simulink model "BaseEngineController_LS"  (Simulink 7.7)
settings: Solver=FixedStepDiscrete  StartTime=0.0  StopTime=10.0  RelTol=1e-3
PreLoadFcn:
  | try, eval([bdroot '_setup']); catch, eval('model_setup', ''); end
InitFcn:
  | try, eval([bdroot '_setup']); catch, eval('model_setup', ''); end
undefined symbols (not defined in the file): ECU555, High, motohawk_build_version, motohawk_trunc_name, motohawk_vardec_config_group, motohawk_vardec_path, True
libraries: MotoHawk_lib x1418, motohawk_control_primitives_lib x183, motohawk_engine_lib x32, simulink x21, motohawk_annotations_lib x9, AutoDoc_lib x8, simulink_extras x4, motohawk_ccp_examples_lib x1, motohawk_control_primitives_motoshare_lib x1
(part 18 of 27)

== system BaseEngineController_LS/Foreground/Inputs/PotentiometerSensors/APP2ForcedAdapt/Function-Call Subsystem ==
  function : TriggerPort  TriggerType=function-call
  First Time : motohawk_control_primitives_lib/First Time  SystemSampleTime=-1
  Logical Operator : Logic  Operator=OR  AllPortsSameDT=off  OutDataTypeStr=boolean
  motohawk_calibration : MotoHawk_lib/Calibration & Probing Blocks/motohawk_calibration  nam='APP2_AlwaysAdapt'  val=0  storage=Calibration  show_more=on  name_source=Use Parameter  data_type=boolean  read_level=1  write_level=1  ovr_cals=on  view_as=Enumeration  enum_struct={'Disabled', 'Enabled'}  vector_style=Wide Row  use_help_units=off  help=''  units=''  use_header_enum=off  row_header_enum={}  col_header_enum={}  use_min_max=off  min_val=-inf  max_val=inf  use_precision=off  precision=''  gain=1  offset=0  exp=1  use_mototune_group=off  mototune_group=motohawk_vardec_path(gcb)
  Out1 : Outport  InitialOutput=false
  wires:
  First Time/1 -> Logical Operator/1
  motohawk_calibration/1 -> Logical Operator/2
  Logical Operator/1 -> Out1/1

== system BaseEngineController_LS/Foreground/Outputs/AEM Infinity Dash/Dash Message 1/RPM_Filt ==
  Raw : Inport
  Constant : Constant
  First Order Low Pass (Tunable) : motohawk_control_primitives_lib/First Order Low Pass (Tunable)  SystemSampleTime=-1  nam='RPMFilt_LowPass'  samp_time=-1  group=motohawk_vardec_path(gcb)
  MinMax : MinMax  Function=max  Inputs=2
  Product : Product  Inputs=*/  RndMeth=Zero
  Product1 : Product  RndMeth=Zero
  Rounding Function : Rounding  Operator=round
  Switch : Switch  Threshold=1
  motohawk_calibration : MotoHawk_lib/Calibration & Probing Blocks/motohawk_calibration  nam='RPMFilt_Enable'  val=0  storage=Calibration  show_more=on  name_source=Use Parameter  data_type=uint8  read_level=1  write_level=1  ovr_cals=on  view_as=Enumeration  enum_struct={'Disabled', 'Enabled'}  vector_style=Wide Row  use_help_units=off  help=''  units=''  use_header_enum=off  row_header_enum={}  col_header_enum={}  use_min_max=off  min_val=-inf  max_val=inf  use_precision=off  precision=''  gain=1  offset=0  exp=1  use_mototune_group=off  mototune_group=motohawk_vardec_path(gcb)
  motohawk_calibration1 : MotoHawk_lib/Calibration & Probing Blocks/motohawk_calibration  nam='RPMFilt_RoundValue'  val=10  storage=Calibration  show_more=on  name_source=Use Parameter  data_type=uint16  read_level=1  write_level=1  ovr_cals=on  view_as=Number  enum_struct={'Disabled', 'Enabled'}  vector_style=Wide Row  use_help_units=on  help='RPM round value'  units='RPM'  use_header_enum=off  row_header_enum={}  col_header_enum={}  use_min_max=on  min_val=0  max_val=1000  use_precision=off  precision=''  gain=1  offset=0  exp=1  use_mototune_group=off  mototune_group=motohawk_vardec_path(gcb)
  motohawk_probe : MotoHawk_lib/Calibration & Probing Blocks/motohawk_probe  nam='RPMFilt_Final'  show_more=off  name_source=Use Parameter  read_level=1  view_as=Number  enum_struct={'Disabled', 'Enabled'}  vector_style=Wide Row  use_help_units=off  help=''  units=''  use_header_enum=off  row_header_enum={}  col_header_enum={}  use_precision=off  precision=''  gain=1  offset=0  exp=1  use_mototune_group=off  mototune_group=motohawk_vardec_path(gcb)
  motohawk_probe1 : MotoHawk_lib/Calibration & Probing Blocks/motohawk_probe  nam='RPMFilt_PostLowPass'  show_more=off  name_source=Use Parameter  read_level=1  view_as=Number  enum_struct={'Disabled', 'Enabled'}  vector_style=Wide Row  use_help_units=off  help=''  units=''  use_header_enum=off  row_header_enum={}  col_header_enum={}  use_precision=off  precision=''  gain=1  offset=0  exp=1  use_mototune_group=off  mototune_group=motohawk_vardec_path(gcb)
  Filt : Outport
  wires:
  Switch/1 -> Filt/1, motohawk_probe/1
  Raw/1 -> Switch/3, [RPM]
  motohawk_calibration/1 -> Switch/2
  Constant/1 -> MinMax/2
  motohawk_calibration1/1 -> MinMax/1
  MinMax/1 -> Product/2, Product1/2
  Product/1 -> Rounding Function/1
  Rounding Function/1 -> Product1/1
  Product1/1 -> Switch/1
  [RPM] -> First Order Low Pass (Tunable)/1
  First Order Low Pass (Tunable)/1 -> Product/1, motohawk_probe1/1

== system BaseEngineController_LS/Foreground/Outputs/AEM Infinity Dash/Dash Message 2/PHI_Filt ==
  PHI RAW : Inport
  PHI DR : Inport  Port=2
  Constant : Constant
  DecreasingFilter : Subsystem  TreatAsAtomicUnit=on
  First Order Low Pass : motohawk_control_primitives_lib/First Order Low Pass  SystemSampleTime=-1
  IncreasingFilter : Subsystem  TreatAsAtomicUnit=on
  Merge : Merge
  MinMax : MinMax  Function=max  Inputs=2  SaturateOnIntegerOverflow=on  InputSameDT=on
  Product : Product  Inputs=*/  SaturateOnIntegerOverflow=on  InputSameDT=on  OutDataTypeStr=Inherit: Same as first input
  Relational Operator3 : RelationalOperator  Operator=>  OutDataTypeStr=boolean
  Relational Operator4 : RelationalOperator  Operator=<  OutDataTypeStr=boolean
  Switch : Switch  Threshold=1
  Switch1 : Switch  Threshold=1
  Unit Delay{1..5} (5 alike) : UnitDelay  SampleTime=-1
  motohawk_calibration : MotoHawk_lib/Calibration & Probing Blocks/motohawk_calibration  nam='PHI1_DefaultVal'  val=0.5  storage=Calibration  show_more=off  name_source=Use Parameter  data_type=Inherit from 'Default Value'  read_level=1  write_level=1  ovr_cals=on  view_as=Number  enum_struct={'Disabled', 'Enabled'}  vector_style=Wide Row  use_help_units=off  help=''  units=''  use_header_enum=off  row_header_enum={}  col_header_enum={}  use_min_max=off  min_val=-inf  max_val=inf  use_precision=off  precision=''  gain=1  offset=0  exp=1  use_mototune_group=off  mototune_group=motohawk_vardec_path(gcb)
  motohawk_delta_time : MotoHawk_lib/Extra Development Blocks/motohawk_delta_time  samp_time=.005  init_val=.005  mode=Seconds (double)
  motohawk_probe : MotoHawk_lib/Calibration & Probing Blocks/motohawk_probe  nam='PHI1_FiltFin'  show_more=off  name_source=Use Parameter  read_level=1  view_as=Number  enum_struct={'Disabled', 'Enabled'}  vector_style=Wide Row  use_help_units=off  help=''  units=''  use_header_enum=off  row_header_enum={}  col_header_enum={}  use_precision=off  precision=''  gain=1  offset=0  exp=1  use_mototune_group=off  mototune_group=motohawk_vardec_path(gcb)
  Filt Out : Outport
  wires:
  PHI DR/1 -> Unit Delay5/1
  motohawk_calibration/1 -> Switch/3
  Unit Delay4/1 -> Unit Delay3/1
  Unit Delay3/1 -> Unit Delay1/1
  Unit Delay1/1 -> Unit Delay2/1
  Unit Delay2/1 -> Relational Operator4/1, Relational Operator3/1
  motohawk_delta_time/1 -> MinMax/1, Product/1
  MinMax/1 -> Product/2
  Merge/1 -> MinMax/2
  Relational Operator4/1 -> IncreasingFilter/Enable
  Relational Operator3/1 -> DecreasingFilter/Enable
  DecreasingFilter/1(Out1) -> Merge/2
  IncreasingFilter/1(Out1) -> Merge/1
  PHI RAW/1 -> First Order Low Pass/1, Unit Delay4/1, Relational Operator3/2, Relational Operator4/2
  [PHI_DR] -> Switch1/2
  Product/1 -> Switch1/1
  Constant/1 -> Switch1/3
  Switch1/1 -> First Order Low Pass/2
  First Order Low Pass/1 -> Switch/1
  Switch/1 -> Filt Out/1, motohawk_probe/1
  Unit Delay5/1 -> Switch/2, [PHI_DR]

== system BaseEngineController_LS/Foreground/Outputs/AEM Infinity Dash/Dash Message 2/PHI_Filt1 ==
  PHI RAW : Inport
  PHI DR : Inport  Port=2
  Constant : Constant
  DecreasingFilter : Subsystem  TreatAsAtomicUnit=on
  First Order Low Pass : motohawk_control_primitives_lib/First Order Low Pass  SystemSampleTime=-1
  IncreasingFilter : Subsystem  TreatAsAtomicUnit=on
  Merge : Merge
  MinMax : MinMax  Function=max  Inputs=2  SaturateOnIntegerOverflow=on  InputSameDT=on
  Product : Product  Inputs=*/  SaturateOnIntegerOverflow=on  InputSameDT=on  OutDataTypeStr=Inherit: Same as first input
  Relational Operator3 : RelationalOperator  Operator=>  OutDataTypeStr=boolean
  Relational Operator4 : RelationalOperator  Operator=<  OutDataTypeStr=boolean
  Switch : Switch  Threshold=1
  Switch1 : Switch  Threshold=1
  Unit Delay{1..5} (5 alike) : UnitDelay  SampleTime=-1
  motohawk_calibration : MotoHawk_lib/Calibration & Probing Blocks/motohawk_calibration  nam='PHI2_DefaultVal'  val=0.5  storage=Calibration  show_more=off  name_source=Use Parameter  data_type=Inherit from 'Default Value'  read_level=1  write_level=1  ovr_cals=on  view_as=Number  enum_struct={'Disabled', 'Enabled'}  vector_style=Wide Row  use_help_units=off  help=''  units=''  use_header_enum=off  row_header_enum={}  col_header_enum={}  use_min_max=off  min_val=-inf  max_val=inf  use_precision=off  precision=''  gain=1  offset=0  exp=1  use_mototune_group=off  mototune_group=motohawk_vardec_path(gcb)
  motohawk_delta_time : MotoHawk_lib/Extra Development Blocks/motohawk_delta_time  samp_time=.005  init_val=.005  mode=Seconds (double)
  motohawk_probe : MotoHawk_lib/Calibration & Probing Blocks/motohawk_probe  nam='PHI2_FiltFin'  show_more=off  name_source=Use Parameter  read_level=1  view_as=Number  enum_struct={'Disabled', 'Enabled'}  vector_style=Wide Row  use_help_units=off  help=''  units=''  use_header_enum=off  row_header_enum={}  col_header_enum={}  use_precision=off  precision=''  gain=1  offset=0  exp=1  use_mototune_group=off  mototune_group=motohawk_vardec_path(gcb)
  Filt Out : Outport
  wires:
  PHI DR/1 -> Unit Delay5/1
  motohawk_calibration/1 -> Switch/3
  Unit Delay4/1 -> Unit Delay3/1
  Unit Delay3/1 -> Unit Delay1/1
  Unit Delay1/1 -> Unit Delay2/1
  Unit Delay2/1 -> Relational Operator4/1, Relational Operator3/1
  motohawk_delta_time/1 -> MinMax/1, Product/1
  MinMax/1 -> Product/2
  Merge/1 -> MinMax/2
  Relational Operator4/1 -> IncreasingFilter/Enable
  Relational Operator3/1 -> DecreasingFilter/Enable
  DecreasingFilter/1(Out1) -> Merge/2
  IncreasingFilter/1(Out1) -> Merge/1
  PHI RAW/1 -> First Order Low Pass/1, Unit Delay4/1, Relational Operator3/2, Relational Operator4/2
  [PHI_DR] -> Switch1/2
  Product/1 -> Switch1/1
  Constant/1 -> Switch1/3
  Switch1/1 -> First Order Low Pass/2
  First Order Low Pass/1 -> Switch/1
  Switch/1 -> Filt Out/1, motohawk_probe/1
  Unit Delay5/1 -> Switch/2, [PHI_DR]

== system BaseEngineController_LS/Foreground/Outputs/Coil Control/Coil Enable Manager/EST Enable TDC Counter ==
  CrankCounter : UnitDelay  SampleTime=-1
  Data Type Conversion : DataTypeConversion  OutDataTypeStr=int8
  EST Enable TDC Counter Stateflow : Stateflow chart  TreatAsAtomicUnit=on
  Relational Operator1 : RelationalOperator  OutDataTypeStr=boolean
  TDC_Counter : Subsystem  TreatAsAtomicUnit=on
  motohawk_calibration1 : MotoHawk_lib/Calibration & Probing Blocks/motohawk_calibration  nam='SparkEnableTDCCounts'  val=0  storage=Calibration  show_more=on  name_source=Use Parameter  data_type=Inherit via back propagation  read_level=1  write_level=1  ovr_cals=on  view_as=Number  enum_struct={'Disabled', 'Enabled'}  vector_style=Wide Row  use_help_units=on  help='Do not enable spark until this many TDCs have occurred in order to guarantee cam synchronization. This number should typically be 2.'  units=''  use_header_enum=off  row_header_enum={}  col_header_enum={}  use_min_max=off  min_val=-inf  max_val=inf  use_precision=off  precision=''  gain=1  offset=0  exp=1  use_mototune_group=on  mototune_group=motohawk_vardec_path(gcb)
  motohawk_data_def : MotoHawk_lib/Data Storage Blocks/motohawk_data_def  nam='TDC'  container_nam=''  data=0  typ=double  struct_nam='MyStruct'  storage=Volatile  outputRef=off  use_vardec=off  window=Display  read_level=1  write_level=1  ovr_cals=on  view_as=Number  enum_struct={'Disabled', 'Enabled'}  vector_style=Wide Row  use_help_units=off  help=''  units=''  use_header_enum=off  row_header_enum=''  col_header_enum=''  use_min_max=off  min_val=-inf  max_val=inf  use_precision=off  precision=''  gain=1  offset=0  exp=1  use_mototune_group=off  mototune_group=motohawk_vardec_path(gcb)  eval_name=MyData  data_stores=motohawk_sfun_data_def_data_stores  struct_instances=motohawk_sfun_data_def_struct_instances  vardecs=motohawk_sfun_data_def_vardecs
  motohawk_data_read : MotoHawk_lib/Data Storage Blocks/motohawk_data_read  source=Lookup By Name  structure=Scalar  operation=Read scalar from location by index  sz_vec=4  sz_row=2  sz_col=3  typ=double  nam='TDC'  checkNull=on  struct_inst_name='MyData'  struct_nam='MyStruct'
  motohawk_data_read3 : MotoHawk_lib/Data Storage Blocks/motohawk_data_read  source=Lookup By Name  structure=Scalar  operation=Read scalar from location by index  sz_vec=4  sz_row=2  sz_col=3  typ=uint8  nam='EngineState'  checkNull=on  struct_inst_name='Struct1'  struct_nam='MyStruct'
  motohawk_data_write : MotoHawk_lib/Data Storage Blocks/motohawk_data_write  source=Lookup By Name  structure=Scalar  operation=Write entire data structure at once  sz_vec=9  sz_row=2  sz_col=9  typ=double  nam='TDC'  checkNull=on  write_read_only=off  struct_inst_name=''  struct_name='MyStruct'
  motohawk_probe1 : MotoHawk_lib/Calibration & Probing Blocks/motohawk_probe  nam='EST_TDCEnabled'  show_more=on  name_source=Use Parameter  read_level=1  view_as=Enumeration  enum_struct={'Disabled', 'Enabled'}  vector_style=Wide Row  use_help_units=on  help=''  units=''  use_header_enum=off  row_header_enum={}  col_header_enum={}  use_precision=off  precision=''  gain=1  offset=0  exp=1  use_mototune_group=on  mototune_group=motohawk_vardec_path(gcb)
  motohawk_probe2 : MotoHawk_lib/Calibration & Probing Blocks/motohawk_probe  nam='TDCCountThreshEnabled'  show_more=on  name_source=Use Parameter  read_level=1  view_as=Enumeration  enum_struct={'Disabled', 'Enabled'}  vector_style=Wide Row  use_help_units=on  help=''  units=''  use_header_enum=off  row_header_enum={}  col_header_enum={}  use_precision=off  precision=''  gain=1  offset=0  exp=1  use_mototune_group=on  mototune_group=motohawk_vardec_path(gcb)
  motohawk_probe3 : MotoHawk_lib/Calibration & Probing Blocks/motohawk_probe  nam='TDCCount'  show_more=on  name_source=Use Parameter  read_level=1  view_as=Number  enum_struct={'Disabled', 'Enabled'}  vector_style=Wide Row  use_help_units=on  help="'Number of TDC events counted after stall.  This will reset once in Crank and Run.'"  units=''  use_header_enum=off  row_header_enum={}  col_header_enum={}  use_precision=off  precision=''  gain=1  offset=0  exp=1  use_mototune_group=on  mototune_group=motohawk_vardec_path(gcb)
  motohawk_trigger1 : MotoHawk_lib/Trigger Blocks/motohawk_trigger  Tag=Trigger  trigger=FGND_TDC_EVENT  function_name=Trigger_FGND_TDC_EVENT_5546p0017  priority_order=0  inherited=on  run_disabled=off  override_app_monitor=off  target=ECU555_80
  Enable : Outport
  wires:
  CrankCounter/1 -> TDC_Counter/1(Reset)
  EST Enable TDC Counter Stateflow/1(CounterReset) -> CrankCounter/1
  Relational Operator1/1 -> motohawk_probe2/1, EST Enable TDC Counter Stateflow/1(CounterEnabled)
  TDC_Counter/1(CrankCount) -> motohawk_probe3/1, Relational Operator1/1
  motohawk_data_read3/1 -> EST Enable TDC Counter Stateflow/2(EngineState)
  EST Enable TDC Counter Stateflow/2(ESTEnable) -> Data Type Conversion/1
  motohawk_calibration1/1 -> Relational Operator1/2
  motohawk_trigger1/1 -> TDC_Counter/Trigger
  EST Enable TDC Counter Stateflow/3(StateO) -> motohawk_data_write/1
  motohawk_data_read/1 -> EST Enable TDC Counter Stateflow/3(State)
  Data Type Conversion/1 -> motohawk_probe1/1, Enable/1

== system BaseEngineController_LS/Foreground/Control/ActuatorCharacterization/Electronic Throttle Controller/PID With Damper Terms (Tunable)/DamperSwitch ==
  TPS : Inport
  Filtered Derivative : Subsystem
  Hysterisis : motohawk_control_primitives_lib/Hysterisis  SystemSampleTime=-1
  Relational Operator : RelationalOperator  Operator=>  ZeroCross=off  InputSameDT=on
  Sum1 : Sum  Inputs=+-|
  motohawk_calibration10 : MotoHawk_lib/Calibration & Probing Blocks/motohawk_calibration  nam=[prefix 'DamperSwitchHyst']  val=0  storage=Calibration  show_more=on  name_source=Use Parameter  data_type=Inherit from 'Default Value'  read_level=1  write_level=1  ovr_cals=on  view_as=Number  enum_struct={'Disabled', 'Enabled'}  vector_style=Wide Row  use_help_units=on  help='Hysterisis around the ThrPosDamperSwitchThresh.'  units='%/s'  use_header_enum=off  row_header_enum={}  col_header_enum={}  use_min_max=off  min_val=-inf  max_val=inf  use_precision=off  precision=''  gain=1  offset=0  exp=1  use_mototune_group=on  mototune_group=motohawk_vardec_path(gcb)
  motohawk_calibration5 : MotoHawk_lib/Calibration & Probing Blocks/motohawk_calibration  nam=[prefix 'DamperSwitchThresh']  val=0  storage=Calibration  show_more=on  name_source=Use Parameter  data_type=Inherit from 'Default Value'  read_level=1  write_level=1  ovr_cals=on  view_as=Number  enum_struct={'Disabled', 'Enabled'}  vector_style=Wide Row  use_help_units=on  help='When filtered derivative of TPS is greater than this threshold, Damper_Up gain will be used.'  units='%/s'  use_header_enum=off  row_header_enum={}  col_header_enum={}  use_min_max=off  min_val=-inf  max_val=inf  use_precision=off  precision=''  gain=1  offset=0  exp=1  use_mototune_group=on  mototune_group=motohawk_vardec_path(gcb)
  motohawk_probe1 : MotoHawk_lib/Calibration & Probing Blocks/motohawk_probe  nam=[prefix 'DamperSwtichState']  show_more=on  name_source=Use Parameter  read_level=1  view_as=Number  enum_struct={'Disabled', 'Enabled'}  vector_style=Wide Row  use_help_units=off  help=''  units=''  use_header_enum=off  row_header_enum={}  col_header_enum={}  use_precision=off  precision=''  gain=1  offset=0  exp=1  use_mototune_group=on  mototune_group=motohawk_vardec_path(gcb)
  motohawk_probe2 : MotoHawk_lib/Calibration & Probing Blocks/motohawk_probe  nam=[prefix 'DamperTPSThresh']  show_more=on  name_source=Use Parameter  read_level=1  view_as=Number  enum_struct={'Disabled', 'Enabled'}  vector_style=Wide Row  use_help_units=off  help=''  units=''  use_header_enum=off  row_header_enum={}  col_header_enum={}  use_precision=off  precision=''  gain=1  offset=0  exp=1  use_mototune_group=on  mototune_group=motohawk_vardec_path(gcb)
  motohawk_probe3 : MotoHawk_lib/Calibration & Probing Blocks/motohawk_probe  nam=[prefix 'DamperTPS']  show_more=on  name_source=Use Parameter  read_level=1  view_as=Number  enum_struct={'Disabled', 'Enabled'}  vector_style=Wide Row  use_help_units=off  help=''  units=''  use_header_enum=off  row_header_enum={}  col_header_enum={}  use_precision=off  precision=''  gain=1  offset=0  exp=1  use_mototune_group=on  mototune_group=motohawk_vardec_path(gcb)
  SwitchState : Outport
  wires:
  Hysterisis/1 -> Relational Operator/2, motohawk_probe2/1
  Filtered Derivative/1(Filt_Deriv) -> Relational Operator/1, motohawk_probe3/1, Hysterisis/2
  motohawk_calibration5/1 -> Sum1/1, Hysterisis/1
  motohawk_calibration10/1 -> Sum1/2
  Sum1/1 -> Hysterisis/3
  TPS/1 -> Filtered Derivative/1(Raw)
  Relational Operator/1 -> SwitchState/1, motohawk_probe1/1

== system BaseEngineController_LS/Foreground/Control/ActuatorCharacterization/Electronic Throttle Controller/PID With Damper Terms (Tunable)/IGain ==
  ErrorIdx : Inport
  Product : Product  RndMeth=Zero
  motohawk_calibration2 : MotoHawk_lib/Calibration & Probing Blocks/motohawk_calibration  nam=[prefix 'IGain']  val=50  storage=Calibration  show_more=on  name_source=Use Parameter  data_type=Inherit from 'Default Value'  read_level=1  write_level=1  ovr_cals=on  view_as=Number  enum_struct={'Disabled', 'Enabled'}  vector_style=Wide Row  use_help_units=on  help='PID Integral Gain'  units='mult'  use_header_enum=off  row_header_enum={}  col_header_enum={}  use_min_max=off  min_val=-inf  max_val=inf  use_precision=off  precision=''  gain=1  offset=0  exp=1  use_mototune_group=on  mototune_group=motohawk_vardec_path(gcb)
  motohawk_interpolation_1d : MotoHawk_lib/Lookup Tables/motohawk_interpolation_1d  nam='ETC_IGainMult'  table_data=[.5 .7 1 2 3 3 2 1 .7 .5]  show_more=on  data_type=Inherit from 'Table Data'  storage=NonAdaptive  read_level=1  write_level=1  ovr_cals=on  use_help=on  help='Multiplier on the ETC I gain based on ETC error.'  units=''  use_min_max=off  min_val=-inf  max_val=inf  use_precision=off  precision=''  gain=1  offset=0  exp=1  use_links=off  prelookup_block=''  output_name=''  use_mototune_group=on  mototune_group=motohawk_vardec_path(gcb)
  IGain : Outport
  wires:
  motohawk_calibration2/1 -> Product/2
  motohawk_interpolation_1d/1 -> Product/1
  Product/1 -> IGain/1
  ErrorIdx/1 -> motohawk_interpolation_1d/1

== system BaseEngineController_LS/Foreground/Control/ActuatorCharacterization/Electronic Throttle Controller/PID With Damper Terms (Tunable)/PGain ==
  ErrorIdx : Inport
  Product : Product  RndMeth=Zero
  motohawk_calibration : MotoHawk_lib/Calibration & Probing Blocks/motohawk_calibration  nam=[prefix 'PGain']  val=15  storage=Calibration  show_more=on  name_source=Use Parameter  data_type=Inherit from 'Default Value'  read_level=1  write_level=1  ovr_cals=on  view_as=Number  enum_struct={'Disabled', 'Enabled'}  vector_style=Wide Row  use_help_units=on  help='PID Proportional Gain'  units='mult'  use_header_enum=off  row_header_enum={}  col_header_enum={}  use_min_max=off  min_val=-inf  max_val=inf  use_precision=off  precision=''  gain=1  offset=0  exp=1  use_mototune_group=on  mototune_group=motohawk_vardec_path(gcb)
  motohawk_interpolation_1d : MotoHawk_lib/Lookup Tables/motohawk_interpolation_1d  nam='ETC_PGainMult'  table_data=ones(1,10)  show_more=on  data_type=Inherit from 'Table Data'  storage=NonAdaptive  read_level=1  write_level=1  ovr_cals=on  use_help=on  help='Multiplier on the ETC P gain based on ETC error.'  units=''  use_min_max=off  min_val=-inf  max_val=inf  use_precision=off  precision=''  gain=1  offset=0  exp=1  use_links=off  prelookup_block=''  output_name=''  use_mototune_group=on  mototune_group=motohawk_vardec_path(gcb)
  PGain : Outport
  wires:
  ErrorIdx/1 -> motohawk_interpolation_1d/1
  Product/1 -> PGain/1
  motohawk_interpolation_1d/1 -> Product/1
  motohawk_calibration/1 -> Product/2

== system BaseEngineController_LS/Foreground/Control/ActuatorCharacterization/Electronic Throttle Controller/PID With Damper Terms (Tunable)/PID With Damper Terms ==
  note: Universal PID Controller
      | with Dampers
  Actual : Inport
  SetPt : Inport  Port=2
  k_Err : Inport  Port=3
  k_P : Inport  Port=4
  k_I : Inport  Port=5
  k_D : Inport  Port=6
  k_Dmp,u : Inport  Port=7
  k_Dmp,d : Inport  Port=8
  IC : Inport  Port=9
  I_min : Inport  Port=10
  I_max : Inport  Port=11
  I_reset : Inport  Port=12
  DamperSwitchState : Inport  Port=13
  Data Type Conversion : DataTypeConversion  SaturateOnIntegerOverflow=on  RndMeth=Zero
  Derivitive1 : motohawk_control_primitives_lib/Derivitive  SystemSampleTime=-1  samp_time=.005
  Derivitive3 : motohawk_control_primitives_lib/Derivitive  SystemSampleTime=-1  samp_time=.005
  Integrator : motohawk_control_primitives_lib/Integrator  SystemSampleTime=-1  samp_time=.005
  Model Info : simulink/Model-Wide Utilities/Model Info  SystemSampleTime=-1  InitialBlockCM=None  BlockCM=None  Frame=on  DisplayStringWithTags=|  HorizontalTextAlignment=Center  LeftAlignmentValue=0.5  SourceBlockDiagram=BaseEngineController_LS  TagMaxNumber=20
      | Model Info:
      | Author: Suhre, Poorman
      | %<Created>
      | %<ModifiedDate>
      | Version: %<ModelVersion>
      | MotoTron Confidential
      | and Propietary
  Product{1..5} (5 alike) : Product  InputSameDT=on  OutDataTypeStr=Inherit: Same as first input
  Sum : Sum  Inputs=-|+|+|+  SaturateOnIntegerOverflow=on  InputSameDT=on  OutDataTypeStr=Inherit: Same as first input
  Sum2 : Sum  Inputs=-|+  SaturateOnIntegerOverflow=on  InputSameDT=on  OutDataTypeStr=Inherit: Same as first input
  Switch : Switch  Threshold=1  ZeroCross=off  InputSameDT=on
  Out : Outport
  Err : Outport  Port=2
  P_term : Outport  Port=3
  I_term : Outport  Port=4
  D_term : Outport  Port=5
  Dmp_term : Outport  Port=6
  wires:
  Derivitive1/1 -> Sum/1, Dmp_term/1
  Derivitive3/1 -> Sum/2, D_term/1
  Product4/1 -> Derivitive3/1
  k_D/1 -> Product4/1
  SetPt/1 -> Sum2/2
  Sum2/1 -> Data Type Conversion/1
  Product5/1 -> Product4/2, Product2/2, Product1/1
  IC/1 -> Integrator/3
  Sum/1 -> Out/1
  Integrator/1 -> Sum/4, I_term/1
  Product2/1 -> Sum/3, P_term/1
  Product1/1 -> Integrator/1
  k_I/1 -> Product1/2
  k_P/1 -> Product2/1
  Actual/1 -> Sum2/1, Product3/2
  I_reset/1 -> Integrator/2
  k_Err/1 -> Product5/2
  Data Type Conversion/1 -> Err/1, Product5/1
  I_min/1 -> Integrator/4
  I_max/1 -> Integrator/5
  Switch/1 -> Product3/1
  k_Dmp,d/1 -> Switch/3
  k_Dmp,u/1 -> Switch/1
  Product3/1 -> Derivitive1/1
  DamperSwitchState/1 -> Switch/2

== system BaseEngineController_LS/Foreground/Control/ActuatorCharacterization/Electronic Throttle Controller/Setpoint Manager/PassThrough ==
  In1 : Inport
  Enable : EnablePort  StatesWhenEnabling=reset
  Out1 : Outport  OutputWhenDisabled=reset  InitialOutput=10
  wires:
  In1/1 -> Out1/1

== system BaseEngineController_LS/Foreground/Control/ActuatorCharacterization/Electronic Throttle Controller/Setpoint Manager/Tuning ==
  Setpoint : Inport
  Mux : Mux  Inputs=3
  Sine Wave : Fcn  Expr=u(2)+u(2)*sin(2*pi*u(3)*u(1))
  Sum : Sum  SaturateOnIntegerOverflow=on
  Switch : Switch  Threshold=1  SaturateOnIntegerOverflow=on
  Time Since Enabled (With Input)1 : motohawk_control_primitives_lib/Time Since Enabled (With Input)1  SystemSampleTime=-1  nam='ETC_Tune_Timer'  samp_time=.005  init=0  upperlim=16000
  motohawk_calibration : MotoHawk_lib/Calibration & Probing Blocks/motohawk_calibration  nam='ETCTuneEnable'  val=0  storage=Calibration  show_more=on  name_source=Use Parameter  data_type=boolean  read_level=1  write_level=1  ovr_cals=on  view_as=Enumeration  enum_struct={'Disabled', 'Enabled'}  vector_style=Wide Row  use_help_units=on  help=''  units=''  use_header_enum=off  row_header_enum={}  col_header_enum={}  use_min_max=off  min_val=-inf  max_val=inf  use_precision=off  precision=''  gain=1  offset=0  exp=1  use_mototune_group=on  mototune_group=motohawk_vardec_path(gcb)
  motohawk_calibration1 : MotoHawk_lib/Calibration & Probing Blocks/motohawk_calibration  nam='ETCTuneFreq'  val=0  storage=Calibration  show_more=on  name_source=Use Parameter  data_type=Inherit from 'Default Value'  read_level=1  write_level=1  ovr_cals=on  view_as=Number  enum_struct={'Disabled', 'Enabled'}  vector_style=Wide Row  use_help_units=on  help=''  units='Hz'  use_header_enum=off  row_header_enum={}  col_header_enum={}  use_min_max=on  min_val=0  max_val=100  use_precision=off  precision=''  gain=1  offset=0  exp=1  use_mototune_group=on  mototune_group=motohawk_vardec_path(gcb)
  motohawk_calibration2 : MotoHawk_lib/Calibration & Probing Blocks/motohawk_calibration  nam='ETCTuneAmp'  val=0  storage=Calibration  show_more=on  name_source=Use Parameter  data_type=Inherit from 'Default Value'  read_level=1  write_level=1  ovr_cals=on  view_as=Number  enum_struct={'Disabled', 'Enabled'}  vector_style=Wide Row  use_help_units=off  help=''  units=''  use_header_enum=off  row_header_enum={}  col_header_enum={}  use_min_max=off  min_val=-inf  max_val=inf  use_precision=off  precision=''  gain=1  offset=0  exp=1  use_mototune_group=on  mototune_group=motohawk_vardec_path(gcb)
  motohawk_calibration4 : MotoHawk_lib/Calibration & Probing Blocks/motohawk_calibration  nam='ETCTuneOffset'  val=0  storage=Calibration  show_more=on  name_source=Use Parameter  data_type=Inherit from 'Default Value'  read_level=1  write_level=1  ovr_cals=on  view_as=Number  enum_struct={'Disabled', 'Enabled'}  vector_style=Wide Row  use_help_units=on  help=''  units=''  use_header_enum=off  row_header_enum={}  col_header_enum={}  use_min_max=off  min_val=-inf  max_val=inf  use_precision=off  precision=''  gain=1  offset=0  exp=1  use_mototune_group=on  mototune_group=motohawk_vardec_path(gcb)
  motohawk_override_abs : MotoHawk_lib/Calibration & Probing Blocks/motohawk_override_abs  SystemSampleTime=-1  parent_name='ETCReq'  parent_val=0  show_more=on  name_source=Use Parameter  parent_read_level=1  parent_override_level=1  view_as=Number  enum_struct={'Disabled', 'Enabled'}  use_help_units=on  parent_help='Override the electronic throttle position'  parent_units='%'  use_min_max=on  parent_min=0  parent_max=100  use_precision=off  parent_precision=''  parent_gain=1  parent_offset=0  parent_exp=1  use_mototune_group=on  parent_group=motohawk_vardec_path(gcb)
  SetpointOut : Outport
  wires:
  Setpoint/1 -> motohawk_override_abs/1
  Switch/1 -> SetpointOut/1
  motohawk_calibration/1 -> Time Since Enabled (With Input)1/1, Switch/2
  Time Since Enabled (With Input)1/1 -> Mux/1
  motohawk_calibration2/1 -> Mux/2
  motohawk_calibration1/1 -> Mux/3
  Mux/1 -> Sine Wave/1
  Sine Wave/1 -> Sum/1
  Sum/1 -> Switch/1
  motohawk_calibration4/1 -> Sum/2
  motohawk_override_abs/1 -> Switch/3

== system BaseEngineController_LS/Foreground/Control/ActuatorCharacterization/Electronic Throttle Controller/Setpoint Manager/Variable Rate Limiter ==
  note: Rate Limiter - Limit allowable change in signal per timestep
  input : Inport
  rise rate : Inport  Port=2
  fall rate : Inport  Port=3
  Product : Product  SaturateOnIntegerOverflow=on  InputSameDT=on  OutDataTypeStr=Inherit: Same as first input
  Product1 : Product  Inputs=/*  SaturateOnIntegerOverflow=on  InputSameDT=on  OutDataTypeStr=Inherit: Same as first input
  Saturation : motohawk_control_primitives_lib/Saturation  SystemSampleTime=-1
  Sum2 : Sum  Inputs=|++  SaturateOnIntegerOverflow=on  InputSameDT=on  OutDataTypeStr=Inherit: Same as first input
  Sum3 : Sum  Inputs=|+-  SaturateOnIntegerOverflow=on  InputSameDT=on  OutDataTypeStr=Inherit: Same as first input
  Unit Delay : UnitDelay  SampleTime=-1
  motohawk_delta_time : MotoHawk_lib/Extra Development Blocks/motohawk_delta_time  samp_time=-1  init_val=0.005  mode=Seconds (double)
  output : Outport  InitialOutput=0
  wires:
  Saturation/1 -> Product/2
  input/1 -> Sum3/1
  Product1/1 -> Saturation/1  "Slope"
  Unit Delay/1 -> Sum3/2, Sum2/2
  Sum2/1 -> Unit Delay/1, output/1
  Product/1 -> Sum2/1
  fall rate/1 -> Saturation/2  "Lo Lim"
  rise rate/1 -> Saturation/3  "Hi Lim"
  Sum3/1 -> Product1/2
  motohawk_delta_time/1 -> Product1/1, Product/1

== system BaseEngineController_LS/Foreground/Control/ActuatorCharacterization/Electronic Throttle Controller/State  Manager/Reset TasksComplete To False ==
  Trigger : TriggerPort
  Constant2 : Constant  Value=false  SampleTime=-1
  motohawk_data_write : MotoHawk_lib/Data Storage Blocks/motohawk_data_write  source=Lookup By Name  structure=Scalar  operation=Write entire data structure at once  sz_vec=-1  sz_row=3  sz_col=2  typ=boolean  nam='ShutDownTasksComplete'  checkNull=off  write_read_only=off  struct_inst_name='Struct1'  struct_name='MyStruct'
  wires:
  Constant2/1 -> motohawk_data_write/1

== system BaseEngineController_LS/Foreground/Control/ActuatorCharacterization/SequenceCutPattern/Hard Cycle Cut Pattern/Cycle1CutPatter ==
  Mux1 : Mux  Inputs=8
  motohawk_calibration10 : MotoHawk_lib/Calibration & Probing Blocks/motohawk_calibration  nam='HardCycle1Cyl4'  val=1  storage=Calibration  show_more=on  name_source=Use Parameter  data_type=int8  read_level=1  write_level=1  ovr_cals=on  view_as=Enumeration  enum_struct={'Enable', 'Cut'}  vector_style=Wide Row  use_help_units=on  help=''  units=''  use_header_enum=off  row_header_enum={}  col_header_enum={}  use_min_max=off  min_val=-inf  max_val=inf  use_precision=off  precision=''  gain=1  offset=0  exp=1  use_mototune_group=on  mototune_group=motohawk_vardec_path(gcb)
  motohawk_calibration11 : MotoHawk_lib/Calibration & Probing Blocks/motohawk_calibration  nam='HardCycle1Cyl1'  val=0  storage=Calibration  show_more=on  name_source=Use Parameter  data_type=int8  read_level=1  write_level=1  ovr_cals=on  view_as=Enumeration  enum_struct={'Enable', 'Cut'}  vector_style=Wide Row  use_help_units=on  help=''  units=''  use_header_enum=off  row_header_enum={}  col_header_enum={}  use_min_max=off  min_val=-inf  max_val=inf  use_precision=off  precision=''  gain=1  offset=0  exp=1  use_mototune_group=on  mototune_group=motohawk_vardec_path(gcb)
  motohawk_calibration12 : MotoHawk_lib/Calibration & Probing Blocks/motohawk_calibration  nam='HardCycle1Cyl5'  val=1  storage=Calibration  show_more=on  name_source=Use Parameter  data_type=int8  read_level=1  write_level=1  ovr_cals=on  view_as=Enumeration  enum_struct={'Enable', 'Cut'}  vector_style=Wide Row  use_help_units=on  help=''  units=''  use_header_enum=off  row_header_enum={}  col_header_enum={}  use_min_max=off  min_val=-inf  max_val=inf  use_precision=off  precision=''  gain=1  offset=0  exp=1  use_mototune_group=on  mototune_group=motohawk_vardec_path(gcb)
  motohawk_calibration13 : MotoHawk_lib/Calibration & Probing Blocks/motohawk_calibration  nam='HardCycle1Cyl6'  val=1  storage=Calibration  show_more=on  name_source=Use Parameter  data_type=int8  read_level=1  write_level=1  ovr_cals=on  view_as=Enumeration  enum_struct={'Enable', 'Cut'}  vector_style=Wide Row  use_help_units=on  help=''  units=''  use_header_enum=off  row_header_enum={}  col_header_enum={}  use_min_max=off  min_val=-inf  max_val=inf  use_precision=off  precision=''  gain=1  offset=0  exp=1  use_mototune_group=on  mototune_group=motohawk_vardec_path(gcb)
  motohawk_calibration14 : MotoHawk_lib/Calibration & Probing Blocks/motohawk_calibration  nam='HardCycle1Cyl7'  val=1  storage=Calibration  show_more=on  name_source=Use Parameter  data_type=int8  read_level=1  write_level=1  ovr_cals=on  view_as=Enumeration  enum_struct={'Enable', 'Cut'}  vector_style=Wide Row  use_help_units=on  help=''  units=''  use_header_enum=off  row_header_enum={}  col_header_enum={}  use_min_max=off  min_val=-inf  max_val=inf  use_precision=off  precision=''  gain=1  offset=0  exp=1  use_mototune_group=on  mototune_group=motohawk_vardec_path(gcb)
  motohawk_calibration15 : MotoHawk_lib/Calibration & Probing Blocks/motohawk_calibration  nam='HardCycle1Cyl8'  val=1  storage=Calibration  show_more=on  name_source=Use Parameter  data_type=int8  read_level=1  write_level=1  ovr_cals=on  view_as=Enumeration  enum_struct={'Enable', 'Cut'}  vector_style=Wide Row  use_help_units=on  help=''  units=''  use_header_enum=off  row_header_enum={}  col_header_enum={}  use_min_max=off  min_val=-inf  max_val=inf  use_precision=off  precision=''  gain=1  offset=0  exp=1  use_mototune_group=on  mototune_group=motohawk_vardec_path(gcb)
  motohawk_calibration8 : MotoHawk_lib/Calibration & Probing Blocks/motohawk_calibration  nam='HardCycle1Cyl2'  val=1  storage=Calibration  show_more=on  name_source=Use Parameter  data_type=int8  read_level=1  write_level=1  ovr_cals=on  view_as=Enumeration  enum_struct={'Enable', 'Cut'}  vector_style=Wide Row  use_help_units=on  help=''  units=''  use_header_enum=off  row_header_enum={}  col_header_enum={}  use_min_max=off  min_val=-inf  max_val=inf  use_precision=off  precision=''  gain=1  offset=0  exp=1  use_mototune_group=on  mototune_group=motohawk_vardec_path(gcb)
  motohawk_calibration9 : MotoHawk_lib/Calibration & Probing Blocks/motohawk_calibration  nam='HardCycle1Cyl3'  val=1  storage=Calibration  show_more=on  name_source=Use Parameter  data_type=int8  read_level=1  write_level=1  ovr_cals=on  view_as=Enumeration  enum_struct={'Enable', 'Cut'}  vector_style=Wide Row  use_help_units=on  help=''  units=''  use_header_enum=off  row_header_enum={}  col_header_enum={}  use_min_max=off  min_val=-inf  max_val=inf  use_precision=off  precision=''  gain=1  offset=0  exp=1  use_mototune_group=on  mototune_group=motohawk_vardec_path(gcb)
  Out : Outport
  wires:
  motohawk_calibration11/1 -> Mux1/1
  motohawk_calibration8/1 -> Mux1/2
  motohawk_calibration9/1 -> Mux1/3
  motohawk_calibration10/1 -> Mux1/4
  motohawk_calibration12/1 -> Mux1/5
  motohawk_calibration13/1 -> Mux1/6
  motohawk_calibration14/1 -> Mux1/7
  motohawk_calibration15/1 -> Mux1/8
  Mux1/1 -> Out/1

== system BaseEngineController_LS/Foreground/Control/ActuatorCharacterization/SequenceCutPattern/Hard Cycle Cut Pattern/Cycle2CutPatter ==
  Mux1 : Mux  Inputs=8
  motohawk_calibration10 : MotoHawk_lib/Calibration & Probing Blocks/motohawk_calibration  nam='HardCycle2Cyl4'  val=1  storage=Calibration  show_more=on  name_source=Use Parameter  data_type=int8  read_level=1  write_level=1  ovr_cals=on  view_as=Enumeration  enum_struct={'Enable', 'Cut'}  vector_style=Wide Row  use_help_units=on  help=''  units=''  use_header_enum=off  row_header_enum={}  col_header_enum={}  use_min_max=off  min_val=-inf  max_val=inf  use_precision=off  precision=''  gain=1  offset=0  exp=1  use_mototune_group=on  mototune_group=motohawk_vardec_path(gcb)
  motohawk_calibration11 : MotoHawk_lib/Calibration & Probing Blocks/motohawk_calibration  nam='HardCycle2Cyl1'  val=1  storage=Calibration  show_more=on  name_source=Use Parameter  data_type=int8  read_level=1  write_level=1  ovr_cals=on  view_as=Enumeration  enum_struct={'Enable', 'Cut'}  vector_style=Wide Row  use_help_units=on  help=''  units=''  use_header_enum=off  row_header_enum={}  col_header_enum={}  use_min_max=off  min_val=-inf  max_val=inf  use_precision=off  precision=''  gain=1  offset=0  exp=1  use_mototune_group=on  mototune_group=motohawk_vardec_path(gcb)
  motohawk_calibration12 : MotoHawk_lib/Calibration & Probing Blocks/motohawk_calibration  nam='HardCycle2Cyl5'  val=1  storage=Calibration  show_more=on  name_source=Use Parameter  data_type=int8  read_level=1  write_level=1  ovr_cals=on  view_as=Enumeration  enum_struct={'Enable', 'Cut'}  vector_style=Wide Row  use_help_units=on  help=''  units=''  use_header_enum=off  row_header_enum={}  col_header_enum={}  use_min_max=off  min_val=-inf  max_val=inf  use_precision=off  precision=''  gain=1  offset=0  exp=1  use_mototune_group=on  mototune_group=motohawk_vardec_path(gcb)
  motohawk_calibration13 : MotoHawk_lib/Calibration & Probing Blocks/motohawk_calibration  nam='HardCycle2Cyl6'  val=1  storage=Calibration  show_more=on  name_source=Use Parameter  data_type=int8  read_level=1  write_level=1  ovr_cals=on  view_as=Enumeration  enum_struct={'Enable', 'Cut'}  vector_style=Wide Row  use_help_units=on  help=''  units=''  use_header_enum=off  row_header_enum={}  col_header_enum={}  use_min_max=off  min_val=-inf  max_val=inf  use_precision=off  precision=''  gain=1  offset=0  exp=1  use_mototune_group=on  mototune_group=motohawk_vardec_path(gcb)
  motohawk_calibration14 : MotoHawk_lib/Calibration & Probing Blocks/motohawk_calibration  nam='HardCycle2Cyl7'  val=1  storage=Calibration  show_more=on  name_source=Use Parameter  data_type=int8  read_level=1  write_level=1  ovr_cals=on  view_as=Enumeration  enum_struct={'Enable', 'Cut'}  vector_style=Wide Row  use_help_units=on  help=''  units=''  use_header_enum=off  row_header_enum={}  col_header_enum={}  use_min_max=off  min_val=-inf  max_val=inf  use_precision=off  precision=''  gain=1  offset=0  exp=1  use_mototune_group=on  mototune_group=motohawk_vardec_path(gcb)
  motohawk_calibration15 : MotoHawk_lib/Calibration & Probing Blocks/motohawk_calibration  nam='HardCycle2Cyl8'  val=1  storage=Calibration  show_more=on  name_source=Use Parameter  data_type=int8  read_level=1  write_level=1  ovr_cals=on  view_as=Enumeration  enum_struct={'Enable', 'Cut'}  vector_style=Wide Row  use_help_units=on  help=''  units=''  use_header_enum=off  row_header_enum={}  col_header_enum={}  use_min_max=off  min_val=-inf  max_val=inf  use_precision=off  precision=''  gain=1  offset=0  exp=1  use_mototune_group=on  mototune_group=motohawk_vardec_path(gcb)
  motohawk_calibration8 : MotoHawk_lib/Calibration & Probing Blocks/motohawk_calibration  nam='HardCycle2Cyl2'  val=0  storage=Calibration  show_more=on  name_source=Use Parameter  data_type=int8  read_level=1  write_level=1  ovr_cals=on  view_as=Enumeration  enum_struct={'Enable', 'Cut'}  vector_style=Wide Row  use_help_units=on  help=''  units=''  use_header_enum=off  row_header_enum={}  col_header_enum={}  use_min_max=off  min_val=-inf  max_val=inf  use_precision=off  precision=''  gain=1  offset=0  exp=1  use_mototune_group=on  mototune_group=motohawk_vardec_path(gcb)
  motohawk_calibration9 : MotoHawk_lib/Calibration & Probing Blocks/motohawk_calibration  nam='HardCycle2Cyl3'  val=1  storage=Calibration  show_more=on  name_source=Use Parameter  data_type=int8  read_level=1  write_level=1  ovr_cals=on  view_as=Enumeration  enum_struct={'Enable', 'Cut'}  vector_style=Wide Row  use_help_units=on  help=''  units=''  use_header_enum=off  row_header_enum={}  col_header_enum={}  use_min_max=off  min_val=-inf  max_val=inf  use_precision=off  precision=''  gain=1  offset=0  exp=1  use_mototune_group=on  mototune_group=motohawk_vardec_path(gcb)
  Out : Outport
  wires:
  Mux1/1 -> Out/1
  motohawk_calibration15/1 -> Mux1/8
  motohawk_calibration14/1 -> Mux1/7
  motohawk_calibration13/1 -> Mux1/6
  motohawk_calibration12/1 -> Mux1/5
  motohawk_calibration10/1 -> Mux1/4
  motohawk_calibration9/1 -> Mux1/3
  motohawk_calibration8/1 -> Mux1/2
  motohawk_calibration11/1 -> Mux1/1

== system BaseEngineController_LS/Foreground/Control/ActuatorCharacterization/SequenceCutPattern/Hard Cycle Cut Pattern/Cycle3CutPatter ==
  Mux1 : Mux  Inputs=8
  motohawk_calibration10 : MotoHawk_lib/Calibration & Probing Blocks/motohawk_calibration  nam='HardCycle3Cyl4'  val=1  storage=Calibration  show_more=on  name_source=Use Parameter  data_type=int8  read_level=1  write_level=1  ovr_cals=on  view_as=Enumeration  enum_struct={'Enable', 'Cut'}  vector_style=Wide Row  use_help_units=on  help=''  units=''  use_header_enum=off  row_header_enum={}  col_header_enum={}  use_min_max=off  min_val=-inf  max_val=inf  use_precision=off  precision=''  gain=1  offset=0  exp=1  use_mototune_group=on  mototune_group=motohawk_vardec_path(gcb)
  motohawk_calibration11 : MotoHawk_lib/Calibration & Probing Blocks/motohawk_calibration  nam='HardCycle3Cyl1'  val=1  storage=Calibration  show_more=on  name_source=Use Parameter  data_type=int8  read_level=1  write_level=1  ovr_cals=on  view_as=Enumeration  enum_struct={'Enable', 'Cut'}  vector_style=Wide Row  use_help_units=on  help=''  units=''  use_header_enum=off  row_header_enum={}  col_header_enum={}  use_min_max=off  min_val=-inf  max_val=inf  use_precision=off  precision=''  gain=1  offset=0  exp=1  use_mototune_group=on  mototune_group=motohawk_vardec_path(gcb)
  motohawk_calibration12 : MotoHawk_lib/Calibration & Probing Blocks/motohawk_calibration  nam='HardCycle3Cyl5'  val=1  storage=Calibration  show_more=on  name_source=Use Parameter  data_type=int8  read_level=1  write_level=1  ovr_cals=on  view_as=Enumeration  enum_struct={'Enable', 'Cut'}  vector_style=Wide Row  use_help_units=on  help=''  units=''  use_header_enum=off  row_header_enum={}  col_header_enum={}  use_min_max=off  min_val=-inf  max_val=inf  use_precision=off  precision=''  gain=1  offset=0  exp=1  use_mototune_group=on  mototune_group=motohawk_vardec_path(gcb)
  motohawk_calibration13 : MotoHawk_lib/Calibration & Probing Blocks/motohawk_calibration  nam='HardCycle3Cyl6'  val=1  storage=Calibration  show_more=on  name_source=Use Parameter  data_type=int8  read_level=1  write_level=1  ovr_cals=on  view_as=Enumeration  enum_struct={'Enable', 'Cut'}  vector_style=Wide Row  use_help_units=on  help=''  units=''  use_header_enum=off  row_header_enum={}  col_header_enum={}  use_min_max=off  min_val=-inf  max_val=inf  use_precision=off  precision=''  gain=1  offset=0  exp=1  use_mototune_group=on  mototune_group=motohawk_vardec_path(gcb)
  motohawk_calibration14 : MotoHawk_lib/Calibration & Probing Blocks/motohawk_calibration  nam='HardCycle3Cyl7'  val=1  storage=Calibration  show_more=on  name_source=Use Parameter  data_type=int8  read_level=1  write_level=1  ovr_cals=on  view_as=Enumeration  enum_struct={'Enable', 'Cut'}  vector_style=Wide Row  use_help_units=on  help=''  units=''  use_header_enum=off  row_header_enum={}  col_header_enum={}  use_min_max=off  min_val=-inf  max_val=inf  use_precision=off  precision=''  gain=1  offset=0  exp=1  use_mototune_group=on  mototune_group=motohawk_vardec_path(gcb)
  motohawk_calibration15 : MotoHawk_lib/Calibration & Probing Blocks/motohawk_calibration  nam='HardCycle3Cyl8'  val=1  storage=Calibration  show_more=on  name_source=Use Parameter  data_type=int8  read_level=1  write_level=1  ovr_cals=on  view_as=Enumeration  enum_struct={'Enable', 'Cut'}  vector_style=Wide Row  use_help_units=on  help=''  units=''  use_header_enum=off  row_header_enum={}  col_header_enum={}  use_min_max=off  min_val=-inf  max_val=inf  use_precision=off  precision=''  gain=1  offset=0  exp=1  use_mototune_group=on  mototune_group=motohawk_vardec_path(gcb)
  motohawk_calibration8 : MotoHawk_lib/Calibration & Probing Blocks/motohawk_calibration  nam='HardCycle3Cyl2'  val=1  storage=Calibration  show_more=on  name_source=Use Parameter  data_type=int8  read_level=1  write_level=1  ovr_cals=on  view_as=Enumeration  enum_struct={'Enable', 'Cut'}  vector_style=Wide Row  use_help_units=on  help=''  units=''  use_header_enum=off  row_header_enum={}  col_header_enum={}  use_min_max=off  min_val=-inf  max_val=inf  use_precision=off  precision=''  gain=1  offset=0  exp=1  use_mototune_group=on  mototune_group=motohawk_vardec_path(gcb)
  motohawk_calibration9 : MotoHawk_lib/Calibration & Probing Blocks/motohawk_calibration  nam='HardCycle3Cyl3'  val=0  storage=Calibration  show_more=on  name_source=Use Parameter  data_type=int8  read_level=1  write_level=1  ovr_cals=on  view_as=Enumeration  enum_struct={'Enable', 'Cut'}  vector_style=Wide Row  use_help_units=on  help=''  units=''  use_header_enum=off  row_header_enum={}  col_header_enum={}  use_min_max=off  min_val=-inf  max_val=inf  use_precision=off  precision=''  gain=1  offset=0  exp=1  use_mototune_group=on  mototune_group=motohawk_vardec_path(gcb)
  Out : Outport
  wires:
  motohawk_calibration11/1 -> Mux1/1
  motohawk_calibration8/1 -> Mux1/2
  motohawk_calibration9/1 -> Mux1/3
  motohawk_calibration10/1 -> Mux1/4
  motohawk_calibration12/1 -> Mux1/5
  motohawk_calibration13/1 -> Mux1/6
  motohawk_calibration14/1 -> Mux1/7
  motohawk_calibration15/1 -> Mux1/8
  Mux1/1 -> Out/1
